simulink model "PID_Controller"  (R2017b)
settings: Solver=VariableStepAuto  StartTime=0.0  StopTime=10.0  RelTol=1e-3  EnableMultiTasking=on
values from neighbouring files (symbols this model uses):
  Fmatrix = [-1/sqrt(2) 0 1/sqrt(2) 1 ... (first row only)    [I_F_matrices.m]
  Imatrix = [1 0 0 1/2 ... (first row only)    [I_F_matrices.m]
libraries: dspmtrx3 x1, dspinverses x1
(part 1 of 5)
settings Model: Creator=as01398  LastModifiedBy=andrewbailey
settings DataIOCC: OutputOption=SpecifiedOutputTimes  OutputTimes=[0:0.2:10]
settings OptimizationCC: LifeSpan=inf
settings DebuggingCC: SFUnexpectedBacktrackingDiag=warning  SFNoUnconditionalDefaultTransitionDiag=warning  SFExecutionAtInitializationDiag=none
settings CodeAppCC: StateflowObjectComments=on
settings GRTTargetCC: TargetLangStandard=C89/C90 (ANSI)  GeneratePreprocessorConditionals=Disable all
settings ConfigComp: CovMetricSettings=dw  CovHtmlReporting=on  CovSaveCumulativeToWorkspaceVar=on  CovSaveSingleToWorkspaceVar=on  CovExternalEMLEnable=off

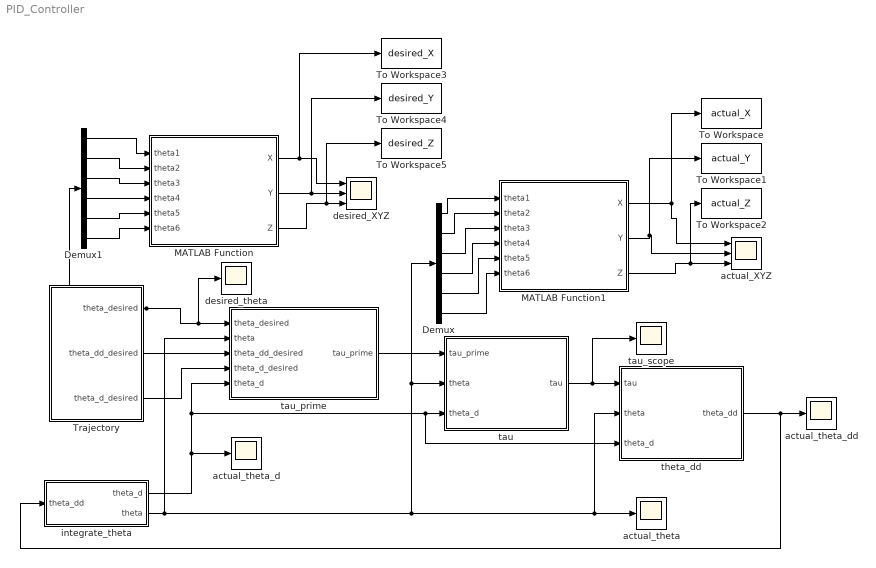
== system PID_Controller ==
  Demux : Demux  Outputs=6
  Demux1 : Demux  Outputs=6
  MATLAB Function : MATLAB Function  TreatAsAtomicUnit=on
  MATLAB Function1 : MATLAB Function  TreatAsAtomicUnit=on
  To Workspace : ToWorkspace  VariableName=actual_X  SampleTime=-1
  To Workspace1 : ToWorkspace  VariableName=actual_Y  SampleTime=-1
  To Workspace2 : ToWorkspace  VariableName=actual_Z  SampleTime=-1
  To Workspace3 : ToWorkspace  VariableName=desired_X  SampleTime=-1
  To Workspace4 : ToWorkspace  VariableName=desired_Y  SampleTime=-1
  To Workspace5 : ToWorkspace  VariableName=desired_Z  SampleTime=-1
  Trajectory : Subsystem
  actual_XYZ : Scope  NumInputPorts=3
  actual_theta : Scope
  actual_theta_d : Scope
  actual_theta_dd : Scope
  desired_XYZ : Scope  NumInputPorts=3
  desired_theta : Scope
  integrate_theta : Subsystem
  tau : Subsystem
  tau_prime : Subsystem
  tau_scope : Scope
  theta_dd : Subsystem
  wires:
  Trajectory/2(theta_dd_desired) -> tau_prime/3(theta_dd_desired)
  Trajectory/3(theta_d_desired) -> tau_prime/4(theta_d_desired)
  tau/1(tau) -> tau_scope/1, theta_dd/1(tau)
  tau_prime/1(tau_prime) -> tau/1(tau_prime)
  theta_dd/1(theta_dd) -> actual_theta_dd/1, integrate_theta/1(theta_dd)
  integrate_theta/2(theta) -> tau_prime/2(theta), Demux/1, tau/2(theta), theta_dd/2(theta), actual_theta/1
  integrate_theta/1(theta_d) -> actual_theta_d/1, theta_dd/3(theta_d), tau/3(theta_d), tau_prime/5(theta_d)
  MATLAB Function1/1(X) -> actual_XYZ/1, To Workspace/1
  Demux1/6 -> MATLAB Function/6(theta6)
  Demux1/3 -> MATLAB Function/3(theta3)
  Demux1/5 -> MATLAB Function/5(theta5)
  Demux1/2 -> MATLAB Function/2(theta2)
  Demux1/1 -> MATLAB Function/1(theta1)
  Demux1/4 -> MATLAB Function/4(theta4)
  MATLAB Function/1(X) -> To Workspace3/1, desired_XYZ/1
  MATLAB Function/2(Y) -> To Workspace4/1, desired_XYZ/2
  MATLAB Function/3(Z) -> To Workspace5/1, desired_XYZ/3
  Trajectory/1(theta_desired) -> desired_theta/1, tau_prime/1(theta_desired), Demux1/1
  MATLAB Function1/2(Y) -> actual_XYZ/2, To Workspace1/1
  MATLAB Function1/3(Z) -> To Workspace2/1, actual_XYZ/3
  Demux/1 -> MATLAB Function1/1(theta1)
  Demux/2 -> MATLAB Function1/2(theta2)
  Demux/3 -> MATLAB Function1/3(theta3)
  Demux/4 -> MATLAB Function1/4(theta4)
  Demux/5 -> MATLAB Function1/5(theta5)
  Demux/6 -> MATLAB Function1/6(theta6)

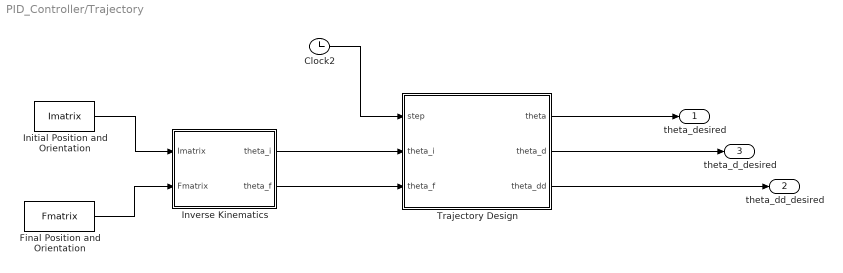
== system PID_Controller/Trajectory ==
  Clock2 : Clock
      settings: Decimation=1000
  Final Position and Orientation : Constant  Value=Fmatrix
  Initial Position and Orientation : Constant  Value=Imatrix
  Inverse Kinematics : MATLAB Function  TreatAsAtomicUnit=on
  Trajectory Design : MATLAB Function  TreatAsAtomicUnit=on
  theta_desired : Outport
  theta_dd_desired : Outport  Port=2
  theta_d_desired : Outport  Port=3
  wires:
  Trajectory Design/3(theta_dd) -> theta_dd_desired/1
  Trajectory Design/2(theta_d) -> theta_d_desired/1
  Trajectory Design/1(theta) -> theta_desired/1
  Inverse Kinematics/2(theta_f) -> Trajectory Design/3(theta_f)
  Inverse Kinematics/1(theta_i) -> Trajectory Design/2(theta_i)
  Final Position and Orientation/1 -> Inverse Kinematics/2(Fmatrix)
  Initial Position and Orientation/1 -> Inverse Kinematics/1(Imatrix)
  Clock2/1 -> Trajectory Design/1(step)

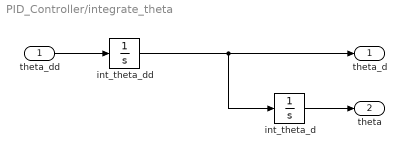
== system PID_Controller/integrate_theta ==
  theta_dd : Inport
  int_theta_d : Integrator
  int_theta_dd : Integrator
  theta_d : Outport
  theta : Outport  Port=2
  wires:
  theta_dd/1 -> int_theta_dd/1
  int_theta_dd/1 -> int_theta_d/1, theta_d/1
  int_theta_d/1 -> theta/1

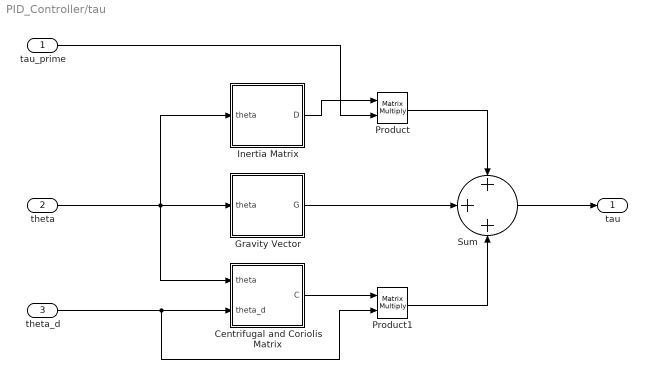
== system PID_Controller/tau ==
  tau_prime : Inport
  theta : Inport  Port=2
  theta_d : Inport  Port=3
  Centrifugal and Coriolis Matrix : Subsystem
  Gravity Vector : Subsystem
  Inertia Matrix : Subsystem
  Product : Product  Multiplication=Matrix(*)
  Product1 : Product  Multiplication=Matrix(*)
  Sum : Sum  Inputs=3
  tau : Outport
  wires:
  theta/1 -> Centrifugal and Coriolis Matrix/1(theta), Gravity Vector/1(theta), Inertia Matrix/1(theta)
  theta_d/1 -> Product1/2, Centrifugal and Coriolis Matrix/2(theta_d)
  Centrifugal and Coriolis Matrix/1(C) -> Product1/1
  Gravity Vector/1(G) -> Sum/2
  Product/1 -> Sum/1
  Product1/1 -> Sum/3
  Sum/1 -> tau/1
  tau_prime/1 -> Product/2
  Inertia Matrix/1(D) -> Product/1

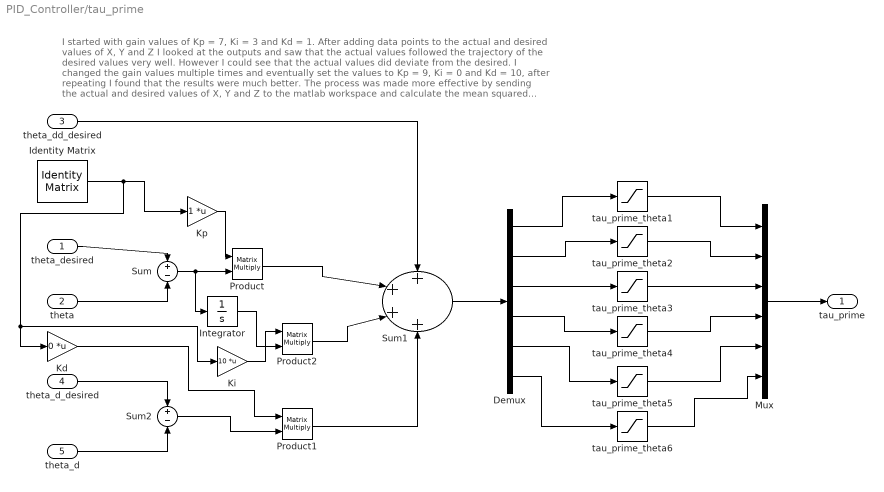
== system PID_Controller/tau_prime ==
  note: I started with gain values of Kp = 7, Ki = 3 and Kd = 1. After adding data points to the actual and desired values of X, Y and Z I looked at the outputs and saw that
      | the actual values followed the trajectory of the desired values very well. However I could see that the actual values did deviate from the desired. I
      | changed the gain values multiple times and eventually set the values to Kp = 9, Ki = 0 and Kd = 10, after repeating I found that the results were much better. The
      | process was made more effective by sending the actual and desired values of X, Y and Z to the matlab workspace and calculate the mean squared error and change
      | the gain values accordingly, I eventually settled with gain values of 0, 0 and 8. This method was highly inaccurate though, therefore I devised a function that would
      | automatically update the gain values in order to obtain the optimal solution, this provided gain values of 2, 0 and 9 which was actually very close to my inital testing.
  theta_desired : Inport
  theta : Inport  Port=2
  theta_dd_desired : Inport  Port=3
  theta_d_desired : Inport  Port=4
  theta_d : Inport  Port=5
  Demux : Demux  Outputs=6
  Identity Matrix : dspmtrx3/Identity Matrix  Inherit=off  N=6  Ts=100  dataType=double  isSigned=on  wordLen=16  udDataType=sfix(16)  fracBitsMode=Best precision  numFracBits=15  OutDataTypeStr=double  LastOutDataTypeStr=double
      settings: SourceProductName=DSP System Toolbox
  Integrator : Integrator
  Kd : Gain  Gain=0  Multiplication=Matrix(K*u)
  Ki : Gain  Gain=10  Multiplication=Matrix(K*u)
  Kp : Gain  Multiplication=Matrix(K*u)
  Mux : Mux  Inputs=6
  Product : Product  Multiplication=Matrix(*)
  Product1 : Product  Multiplication=Matrix(*)
  Product2 : Product  Multiplication=Matrix(*)
  Sum : Sum  Inputs=+-
  Sum1 : Sum  Inputs=++++
  Sum2 : Sum  Inputs=+-
  tau_prime_theta1 : Saturate  UpperLimit=16  LowerLimit=-16
  tau_prime_theta2 : Saturate  UpperLimit=32  LowerLimit=-32
  tau_prime_theta3 : Saturate  UpperLimit=21  LowerLimit=-21
  tau_prime_theta4 : Saturate  UpperLimit=5  LowerLimit=-5
  tau_prime_theta5 : Saturate  UpperLimit=5  LowerLimit=-5
  tau_prime_theta6 : Saturate  UpperLimit=4  LowerLimit=-4
  tau_prime : Outport
  wires:
  theta/1 -> Sum/2
  theta_desired/1 -> Sum/1
  Sum/1 -> Integrator/1, Product/2
  theta_d_desired/1 -> Sum2/1
  theta_d/1 -> Sum2/2
  theta_dd_desired/1 -> Sum1/1
  Sum1/1 -> Demux/1
  Demux/1 -> tau_prime_theta1/1
  Demux/2 -> tau_prime_theta2/1
  Demux/3 -> tau_prime_theta3/1
  Demux/4 -> tau_prime_theta4/1
  Demux/5 -> tau_prime_theta5/1
  Demux/6 -> tau_prime_theta6/1
  tau_prime_theta1/1 -> Mux/1
  tau_prime_theta2/1 -> Mux/2
  tau_prime_theta3/1 -> Mux/3
  tau_prime_theta4/1 -> Mux/4
  tau_prime_theta5/1 -> Mux/5
  tau_prime_theta6/1 -> Mux/6
  Mux/1 -> tau_prime/1
  Identity Matrix/1 -> Ki/1, Kd/1, Kp/1
  Kp/1 -> Product/1
  Product/1 -> Sum1/2
  Product1/1 -> Sum1/4
  Sum2/1 -> Product1/2
  Kd/1 -> Product1/1
  Ki/1 -> Product2/1
  Integrator/1 -> Product2/2
  Product2/1 -> Sum1/3

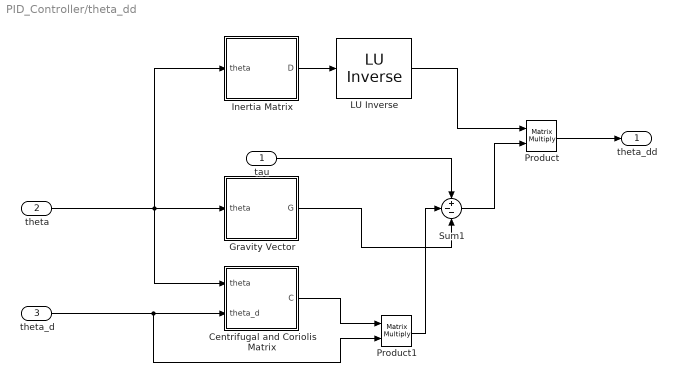
== system PID_Controller/theta_dd ==
  tau : Inport
  theta : Inport  Port=2
  theta_d : Inport  Port=3
  " LU Inverse" : dspinverses/ LU Inverse
      settings: SourceProductName=DSP System Toolbox
  Centrifugal and Coriolis Matrix : Subsystem
  Gravity Vector : Subsystem
  Inertia Matrix : Subsystem
  Product : Product  Multiplication=Matrix(*)
  Product1 : Product  Multiplication=Matrix(*)
  Sum1 : Sum  Inputs=+--
  theta_dd : Outport
  wires:
  theta/1 -> Centrifugal and Coriolis Matrix/1(theta), Gravity Vector/1(theta), Inertia Matrix/1(theta)
  theta_d/1 -> Product1/2, Centrifugal and Coriolis Matrix/2(theta_d)
  Centrifugal and Coriolis Matrix/1(C) -> Product1/1
  Product/1 -> theta_dd/1
  Inertia Matrix/1(D) -> " LU Inverse"/1
  tau/1 -> Sum1/1
  " LU Inverse"/1 -> Product/1
  Sum1/1 -> Product/2
  Product1/1 -> Sum1/2
  Gravity Vector/1(G) -> Sum1/3

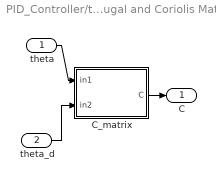
== system PID_Controller/tau/Centrifugal and Coriolis Matrix ==
  theta : Inport
  theta_d : Inport  Port=2
  C_matrix : MATLAB Function  TreatAsAtomicUnit=on
  C : Outport
  wires:
  theta_d/1 -> C_matrix/2(in2)
  theta/1 -> C_matrix/1(in1)
  C_matrix/1(C) -> C/1

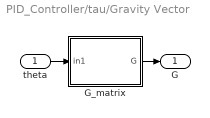
== system PID_Controller/tau/Gravity Vector ==
  theta : Inport
  G_matrix : MATLAB Function  TreatAsAtomicUnit=on
  G : Outport
  wires:
  G_matrix/1(G) -> G/1
  theta/1 -> G_matrix/1(in1)

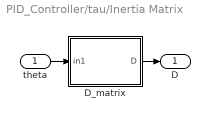
== system PID_Controller/tau/Inertia Matrix ==
  theta : Inport
  D_matrix : MATLAB Function  TreatAsAtomicUnit=on
  D : Outport
  wires:
  D_matrix/1(D) -> D/1
  theta/1 -> D_matrix/1(in1)

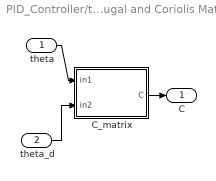
== system PID_Controller/theta_dd/Centrifugal and Coriolis Matrix ==
  theta : Inport
  theta_d : Inport  Port=2
  C_matrix : MATLAB Function  TreatAsAtomicUnit=on
  C : Outport
  wires:
  theta_d/1 -> C_matrix/2(in2)
  theta/1 -> C_matrix/1(in1)
  C_matrix/1(C) -> C/1

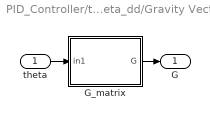
== system PID_Controller/theta_dd/Gravity Vector ==
  theta : Inport
  G_matrix : MATLAB Function  TreatAsAtomicUnit=on
  G : Outport
  wires:
  G_matrix/1(G) -> G/1
  theta/1 -> G_matrix/1(in1)

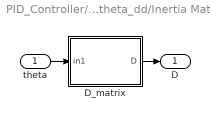
== system PID_Controller/theta_dd/Inertia Matrix ==
  theta : Inport
  D_matrix : MATLAB Function  TreatAsAtomicUnit=on
  D : Outport
  wires:
  D_matrix/1(D) -> D/1
  theta/1 -> D_matrix/1(in1)

== matlab function PID_Controller/MATLAB Function1 ==
  data: theta1 input; X output; theta2 input; theta3 input; theta4 input; theta5 input; theta6 input; Y output; Z output
function [X,Y,Z] = ForwardKinematic(theta1,theta2,theta3,theta4,theta5,theta6)

% Set the variables for the following calculations
a = [0;0.5;0;0;0;0];
d = [0;0.25;0;1;0;0.5];
alpha = [-90;0;90;-90;90;0]*(pi/180);

% Calculate the different A matrices and then calculate the DH matrix
A_1 = A(theta1,a(1),d(1),alpha(1));
A_2 = A(theta2,a(2),d(2),alpha(2));
A_3 = A(theta3,a(3),d(3),alpha(3));
A_4 = A(theta4,a(4),d(4),alpha(4));
A_5 = A(theta5,a(5),d(5),alpha(5));
A_6 = A(theta6,a(6),d(6),alpha(6));

A0_3 = (A_1*A_2)*A_3;
A4_6 = (A_4*A_5)*A_6;

DH = A0_3*A4_6;

% Take the values fo X, Y and Z from the final collumn of the DH matrix
X = DH(1,4);
Y = DH(2,4);
Z = DH(3,4);

end

== matlab function PID_Controller/MATLAB Function ==
  data: theta1 input; X output; theta2 input; theta3 input; theta4 input; theta5 input; theta6 input; Y output; Z output
function [X,Y,Z] = ForwardKinematic(theta1,theta2,theta3,theta4,theta5,theta6)

% Set the variables for the following calculations
a = [0;0.5;0;0;0;0];
d = [0;0.25;0;1;0;0.5];
alpha = [-90;0;90;-90;90;0]*(pi/180);

% Calculate the different A matrices and then calculate the DH matrix
A_1 = A(theta1,a(1),d(1),alpha(1));
A_2 = A(theta2,a(2),d(2),alpha(2));
A_3 = A(theta3,a(3),d(3),alpha(3));
A_4 = A(theta4,a(4),d(4),alpha(4));
A_5 = A(theta5,a(5),d(5),alpha(5));
A_6 = A(theta6,a(6),d(6),alpha(6));

A0_3 = (A_1*A_2)*A_3;
A4_6 = (A_4*A_5)*A_6;

DH = A0_3*A4_6;

% Take the values fo X, Y and Z from the final collumn of the DH matrix
X = DH(1,4);
Y = DH(2,4);
Z = DH(3,4);

end

== matlab function PID_Controller/Trajectory/Inverse Kinematics ==
  data: Imatrix input; theta_i output; theta_f output; Fmatrix input
function [theta_i,theta_f]=IK(Imatrix,Fmatrix)

theta_i=[0;0;0;0;0;0];
theta_f=[0;0;0;0;0;0];
% Initial angles
coder.extrinsic('InverseKinematic')
[qi1,qi2,qi3,qi4,qi5,qi6]=InverseKinematic(Imatrix);
    q01=qi1;
    q02=qi2;
    q03=qi3;
    q04=qi4;
    q05=qi5;
    q06=qi6;
    
% Final angles
[qi1,qi2,qi3,qi4,qi5,qi6]=InverseKinematic(Fmatrix);
    qf1=qi1;
    qf2=qi2;
    qf3=qi3;
    qf4=qi4;
    qf5=qi5;
    qf6=qi6;

theta_i=[q01;q02;q03;q04;q05;q06];
theta_f=[qf1;qf2;qf3;qf4;qf5;qf6];
